simulink model "pneumatic_tank_general"  (R2021a)
settings: Solver=ode15s  StartTime=0.0  StopTime=10  RelTol=1e-4
model workspace (MATLAB code in the model file):
  | V = 0.4; %liter
  | alpha = 1.5/3;
  | p_s = 6; % bar
settings Model: Creator=kjartan  LastModifiedBy=kjartan
settings SolverCC: AlgebraicLoopSolver=TrustRegion
settings DataIOCC: ReturnWorkspaceOutputs=off
settings DebuggingCC: SFMachineParentedDataDiag=warning  ArithmeticOperatorsInVariantConditions=warning
settings SFSimCC: CustomCodeUndefinedFunction=UseInterfaceOnly

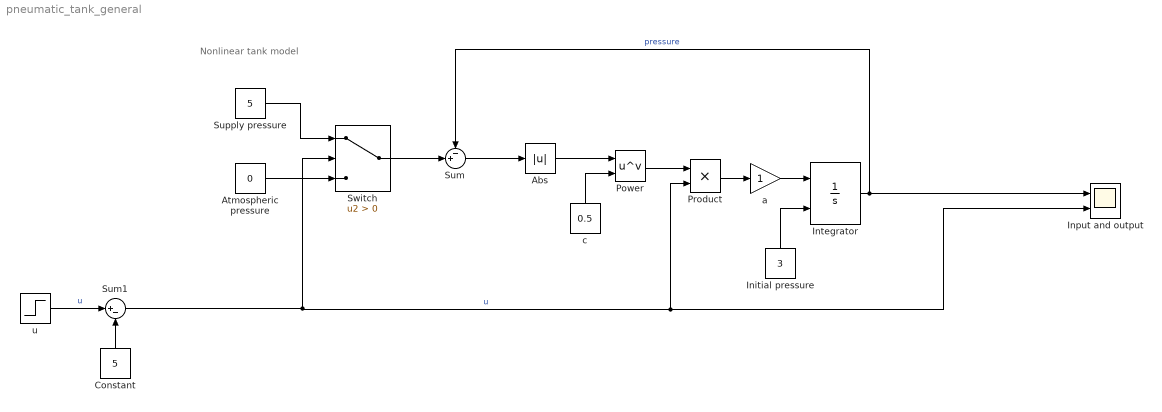
== system pneumatic_tank_general ==
  note: Nonlinear tank model
  Abs : Abs
  Atmospheric pressure : Constant  Value=0
  Constant : Constant  Value=5
  Initial pressure : Constant  Value=3  OutDataTypeStr=Inherit: Inherit via back propagation
  Input and output : Scope  NumInputPorts=2
  Integrator : Integrator  InitialConditionSource=external  InitialCondition=1  LimitOutput=on  UpperSaturationLimit=5  LowerSaturationLimit=0
  Power : Math  Operator=pow  SaturateOnIntegerOverflow=on
  Product : Product
  Sum : Sum  Inputs=-+|
  Sum1 : Sum  Inputs=|+-
  Supply pressure : Constant  Value=5
  Switch : Switch  Criteria=u2 > Threshold
  a : Gain
  c : Constant  Value=0.5
  u : Step  Time=5  Before=4  After=7  SampleTime=0
  wires:
  Integrator/1 -> Sum/1, Input and output/1  "pressure"
  Sum/1 -> Abs/1
  Sum1/1 -> Switch/2, Product/2, Input and output/2  "u"
  a/1 -> Integrator/1
  Product/1 -> a/1
  Supply pressure/1 -> Switch/1
  Atmospheric pressure/1 -> Switch/3
  Switch/1 -> Sum/2
  Power/1 -> Product/1
  Initial pressure/1 -> Integrator/2
  Constant/1 -> Sum1/2
  u/1 -> Sum1/1  "u"
  Abs/1 -> Power/1
  c/1 -> Power/2
